simulink model "linearpll"  (Simulink 6.6)
settings: Solver=ode45  StartTime=0.0  StopTime=50e-6  RelTol=1e-3
libraries: commsynccomp2 x1, dsparch4 x1, dspsnks4 x1
settings Model: Creator=Edwin Pasterkamp  LastModifiedBy=epasterk
settings DebuggingCC: SignalResolutionControl=TryResolveAllWithWarning

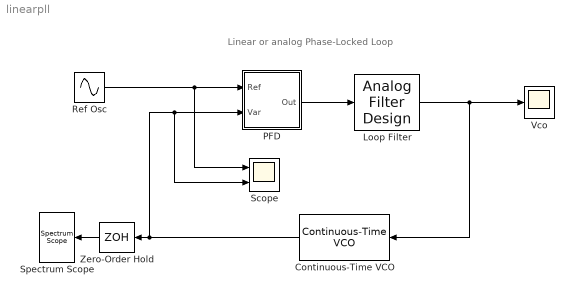
== system linearpll ==
  note: Linear or analog Phase-Locked Loop
  Continuous-Time VCO : commsynccomp2/Continuous-Time VCO  Orientation=left  SystemSampleTime=-1  Ac=1  Fc=1e6  Kc=1e5  Ph=0
  Loop Filter : dsparch4/Analog Filter Design  method=Butterworth  filttype=Lowpass  N=5  Wlo=1e6*2*pi  Whi=80  Rp=1  Rs=180
  PFD : Subsystem
  Ref Osc : Sin  Frequency=2*pi*1e6  SampleTime=0
      settings: AttributesFormatString=%<Frequency> (rad/s)
  Scope : Scope  NumInputPorts=2
      settings: TimeRange=5e-005  YMin=-1.5~-1.5  YMax=1.5~1.5  SaveName=log_linearpll  SampleInput=on  SampleTime=1e-8
  Spectrum Scope : dspsnks4/Spectrum Scope  Orientation=left  DialogController=dspdialog.SpectrumScope  DialogControllerArgs=DataTag0  SystemSampleTime=-1  ScopeProperties=on  Domain=Frequency  HorizSpan=1  UseBuffer=on  BufferSize=512  Overlap=256  inpFftLenInherit=off  FFTlength=512  numAvg=1  DisplayProperties=off  AxisGrid=on  Memory=off  FrameNumber=on  AxisLegend=off  AxisZoom=off  OpenScopeAtSimStart=off  OpenScopeImmediately=off  FigPos=[7 92 1014 145]  AxisProperties=off  XUnits=Hertz  XRange=[0...Fs/2]  InheritXIncr=on  XIncr=1.0  XLabel=Samples  XLimit=Auto  YUnits=dB  XMax=1  XMin=0  YLabel=Magnitude-squared, dB  LineProperties=off  wintypeSpecScope=Kaiser  RsSpecScope=50  betaSpecScope=5  winsampSpecScope=Periodic
      settings: YMin=-67.488756819385  YMax=23.8054648623852
  Vco : Scope
      settings: TimeRange=0.0001  YMin=-1  YMax=1
  Zero-Order Hold : ZeroOrderHold  Orientation=left  SampleTime=1e-7
  wires:
  Ref Osc/1 -> Scope/1, PFD/1(Ref)
  Continuous-Time VCO/1 -> Scope/2, PFD/2(Var), Zero-Order Hold/1
  PFD/1(Out) -> Loop Filter/1
  Loop Filter/1 -> Vco/1, Continuous-Time VCO/1
  Zero-Order Hold/1 -> Spectrum Scope/1

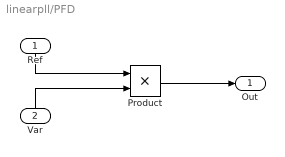
== system linearpll/PFD ==
  Ref : Inport  Orientation=down
  Var : Inport  Orientation=up  Port=2
  Product : Product  RndMeth=Zero
  Out : Outport
  wires:
  Ref/1 -> Product/1
  Var/1 -> Product/2
  Product/1 -> Out/1
